simulink library "zero_cross"  (Simulink 6.3)
undefined symbols (not defined in the file): a, b, bits_to_symb_do, DiscIntNeverNeededParam, do_wait, input_stream_sample, j, lookup_do, offset, sfunpsd2
settings Model: Creator=jon  LastModifiedBy=jwallace  ExtModeAutoUpdateStatusClock=off  StrictBusMsg=None

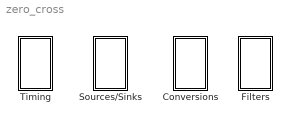
== system zero_cross ==
  Conversions : Subsystem
  Filters : Subsystem
  Sources/Sinks : Subsystem
  "Timing " : Subsystem

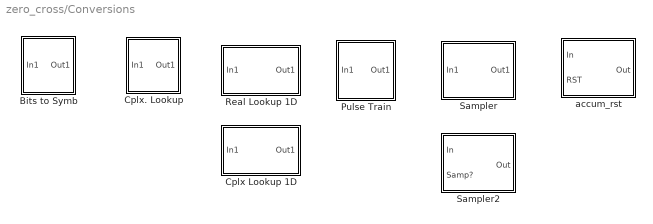
== system zero_cross/Conversions ==
  Bits to Symb : Subsystem
  Cplx Lookup 1D : Subsystem  mask{table=[j -j]}
      mask init:
      | XData = [0:length(table)-1]; YDataRe = real(table); YDataIm = imag(table); XDataEvenlySpacing=1;
  Cplx. Lookup : Subsystem  mask{table=[-1 1]}
      mask help: Does a discrete lookup table.
      mask Help: The table variable has one entry per possible input index.  Note that it is defined to be zero indexed (0 maps to the first table entry, 1 to the second, etc.).
  Pulse Train : Subsystem  mask{period=10}
      mask prompts: period "Period (samples)"
      mask help: Samples the incoming signal and makes a pulse train.
      mask Display: disp(sprintf('T=%d', period));
  Real Lookup 1D : Subsystem  mask{table=[-1 -0.5 0.5 1]}
      mask init:
      | XData = [0:length(table)-1]; YData = table; XDataEvenlySpacing=1;
  Sampler : Subsystem  mask{offset=64, samp_period=10}
      mask prompts: offset "Offset (samples)"; samp_period "Sample Period"
      mask Display: disp(sprintf('del=%d, T=%d', offset, samp_period));
  Sampler2 : Subsystem
  accum_rst : Subsystem

== system zero_cross/Filters ==
  RC FIR Filter : Subsystem  mask{period=10, beta=0.5, root=off, filt_len=128}
      mask prompts: period "Symbol Period"; beta "Roll Off (beta)"; root "Root Filter?"; filt_len "Filter Length (taps)"
      mask init:
      | symb_rate = 1/period; p.fs = symb_rate; p.beta = beta; p.root = root; [h f Ha Hi win] = win_method('rc_filt', p, 1.5*(1+beta)*symb_rate, 1, filt_len, 0); h = h';
      mask Display: plot(f, abs(Ha));
  RECT Filter : Subsystem  AncestorBlock=dsp_blocks/Filters/RC FIR Filter  mask{f0=0.1, f1=0.2, filt_len=64}
      mask prompts: f0 "Low Cutoff (0=LPF)"; f1 "Hi Cutoff"; filt_len "Filter Length (taps)"
      mask init:
      | p.x1 = f0; p.x2 = f0; p.x3 = f1; p.x4 = f1; [h f Ha Hi win] = win_method('pw_lin', p, 0.5, 1, filt_len, 1); h = h';
      mask Display: plot(f, abs(Ha));

== system zero_cross/Sources/Sinks ==
  Averaging Power Spectral Density dB : Subsystem  LoadFcn=sfunpsd2([],[],[],'LoadBlock')  StartFcn=sfunpsd2([],[],[],'Start')  mask(Spectrum Analyzer){npts=128, fftpts=512, HowOften=64, sampleT=1, db_range=20}
      mask prompts: npts "Length of buffer:"; fftpts "Number of points for fft:"; HowOften "Plot after how many points:"; sampleT "Sample time:"; db_range "dB Range:"
      mask help: Spectrum analyzer using graph window.
      mask init:
      | ts=sampleT(1); if length(sampleT) > 1, offset = sampleT(2);, else, offset = 0; end
      settings: CopyFcn=sfunpsd2([],[],[],'CopyBlock')  DeleteFcn=sfunpsd2([],[],[],'DeleteBlock')  NameChangeFcn=sfunpsd2([],[],[],'NameChange')
      mask Help: This block when hooked to the output of a system displays the frequency content of the buffer in the graph window. For more see the M-file sfunpsd.
      mask Display: plot(0,0,100,100,[11,92,92,11,11],[90,90,40,40,90],[82,76,65,57,51,44,35,30,25,20],[65,62,59,63,66,66,67,70,55,50])
  Input Stream : Subsystem  mask{period=10, width=1, fname=data.mat}
      mask prompts: fname "Data Filename"
      mask help: Input Stream: Reads binary data from an input file. Outputs a new value once per period. Width allows you to multiplex output.
      mask init:
      | load(fname); N = floor(length(data)/width); data = reshape(data(1:N*width),width,N);
      mask Help: The function loads the binary data from file fname, which should have a single vector called "data".  The output of the block is updated once every T=width*period.
      mask Display: disp(sprintf('file=%s\nT=%g w=%d', fname, period, width))

== system zero_cross/Timing  ==
  PLL : Subsystem  mask{freq=0.1, freq_out=0.1, phi=0, amp=1, xi=1, K=2, T=200}
      mask prompts: freq "Input Frequency"; freq_out "Output Frequency"; phi "Output Phase"; amp "Output Amplitude"; xi "Damping Factor"; K "Loop Gain"; T "Loop Time Constant (samples)"
      mask help: Implements a phase locked loop (PLL).
      mask init:
      | [a, b, tau1, tau2, Kout] = loop_filter1(T, xi, K);
      mask Display: disp(sprintf('fin=%g fout=%g\nxi=%g Tl=%g\nphi=%g  amp=%g',freq,freq_out,xi,T,phi,amp));
  Real-Time : Subsystem  mask{scale=1}
      mask prompts: scale "Scale Factor"
      mask help: This block slows down a simulation so sample time is some fraction of the real time.
      mask Display: disp('RT');

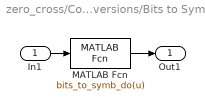
== system zero_cross/Conversions/Bits to Symb ==
  In1 : Inport
  MATLAB Fcn : MATLABFcn  MATLABFcn=bits_to_symb_do(u)  OutputDimensions=1
  Out1 : Outport
  wires:
  MATLAB Fcn/1 -> Out1/1
  In1/1 -> MATLAB Fcn/1

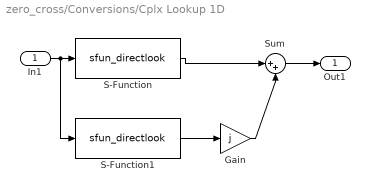
== system zero_cross/Conversions/Cplx Lookup 1D ==
  In1 : Inport
  Gain : Gain  Gain=j  SaturateOnIntegerOverflow=on
  S-Function : S-Function  FunctionName=sfun_directlook  Parameters=XData, YDataRe, XDataEvenlySpacing
  S-Function1 : S-Function  FunctionName=sfun_directlook  Parameters=XData, YDataIm, XDataEvenlySpacing
  Sum : Sum  Inputs=|++  SaturateOnIntegerOverflow=on  InputSameDT=on
  Out1 : Outport
  wires:
  In1/1 -> S-Function1/1, S-Function/1
  S-Function/1 -> Sum/1
  Gain/1 -> Sum/2
  Sum/1 -> Out1/1
  S-Function1/1 -> Gain/1

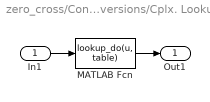
== system zero_cross/Conversions/Cplx. Lookup ==
  In1 : Inport
  MATLAB Fcn : MATLABFcn  MATLABFcn=lookup_do(u, table)  OutputSignalType=complex
  Out1 : Outport
  wires:
  MATLAB Fcn/1 -> Out1/1
  In1/1 -> MATLAB Fcn/1

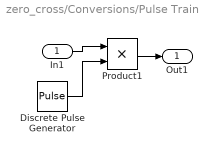
== system zero_cross/Conversions/Pulse Train ==
  In1 : Inport
  Discrete Pulse Generator : DiscretePulseGenerator  Period=period
  Product1 : Product  SaturateOnIntegerOverflow=on  RndMeth=Zero
  Out1 : Outport
  wires:
  Product1/1 -> Out1/1
  In1/1 -> Product1/1
  Discrete Pulse Generator/1 -> Product1/2

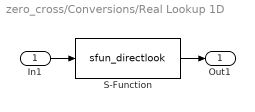
== system zero_cross/Conversions/Real Lookup 1D ==
  In1 : Inport
  S-Function : S-Function  FunctionName=sfun_directlook  Parameters=XData, YData, XDataEvenlySpacing
  Out1 : Outport
  wires:
  S-Function/1 -> Out1/1
  In1/1 -> S-Function/1

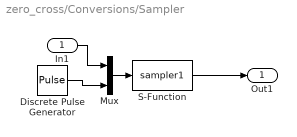
== system zero_cross/Conversions/Sampler ==
  In1 : Inport
  Discrete Pulse Generator : DiscretePulseGenerator  Period=samp_period  PhaseDelay=offset
  Mux : Mux  Inputs=2
  S-Function : S-Function  FunctionName=sampler1
  Out1 : Outport
  wires:
  S-Function/1 -> Out1/1
  Mux/1 -> S-Function/1
  In1/1 -> Mux/1
  Discrete Pulse Generator/1 -> Mux/2

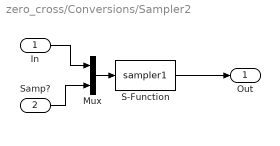
== system zero_cross/Conversions/Sampler2 ==
  In : Inport
  Samp? : Inport  Port=2
  Mux : Mux  Inputs=2
  S-Function : S-Function  FunctionName=sampler1
  Out : Outport
  wires:
  Samp?/1 -> Mux/2
  In/1 -> Mux/1
  Mux/1 -> S-Function/1
  S-Function/1 -> Out/1

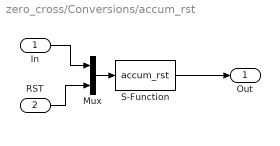
== system zero_cross/Conversions/accum_rst ==
  In : Inport
  RST : Inport  Port=2
  Mux : Mux  Inputs=2
  S-Function : S-Function  FunctionName=accum_rst
  Out : Outport
  wires:
  S-Function/1 -> Out/1
  Mux/1 -> S-Function/1
  In/1 -> Mux/1
  RST/1 -> Mux/2

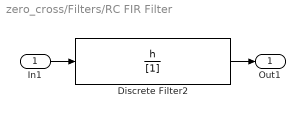
== system zero_cross/Filters/RC FIR Filter ==
  In1 : Inport
  Discrete Filter2 : DiscreteFilter  Numerator=h  Denominator=[1]
  Out1 : Outport
  wires:
  Discrete Filter2/1 -> Out1/1
  In1/1 -> Discrete Filter2/1

== system zero_cross/Filters/RECT Filter ==
  In1 : Inport
  Discrete Filter2 : DiscreteFilter  Numerator=h  Denominator=[1]
  Out1 : Outport
  wires:
  In1/1 -> Discrete Filter2/1
  Discrete Filter2/1 -> Out1/1

== system zero_cross/Sources/Sinks/Averaging Power Spectral Density dB ==
  input signal : Inport
  sfunpsd2 : S-Function  LoadFcn=sfunpsd2([],[],[],'LoadBlock')  StartFcn=sfunpsd2([],[],[],'Start')  FunctionName=sfunpsd2  Parameters=fftpts,npts,HowOften,offset,ts,1,db_range
      settings: CopyFcn=sfunpsd2([],[],[],'CopyBlock')  DeleteFcn=sfunpsd2([],[],[],'DeleteBlock')  NameChangeFcn=sfunpsd2([],[],[],'NameChange')
  wires:
  input signal/1 -> sfunpsd2/1

== system zero_cross/Sources/Sinks/Input Stream ==
  Clock : Clock
  MATLAB Fcn : MATLABFcn  MATLABFcn=input_stream_sample(u, data, period, width)  OutputDimensions=width  Output1D=off
  Out1 : Outport
  wires:
  MATLAB Fcn/1 -> Out1/1
  Clock/1 -> MATLAB Fcn/1

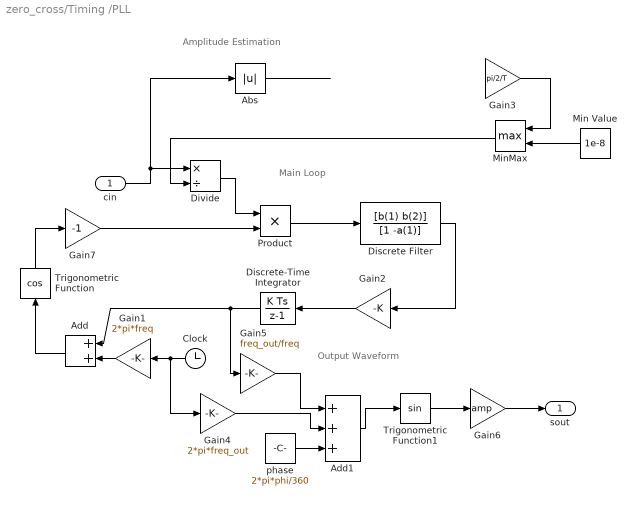
== system zero_cross/Timing /PLL ==
  note: Output Waveform
  note: Main Loop
  note: Amplitude Estimation
  cin : Inport
  Abs : Abs
  Add : Sum  Orientation=left  OutScaling=2^-10
  Add1 : Sum  Inputs=+++  OutScaling=2^-10
  Clock : Clock
  Discrete Filter : DiscreteFilter  Numerator=[b(1) b(2)]  Denominator=[1 -a(1)]
  Discrete-Time Integrator : DiscreteIntegrator  Orientation=left  gainval=1  ICPrevOutput=DiscIntNeverNeededParam  ICPrevScaledInput=DiscIntNeverNeededParam
  Divide : Product  Inputs=*/  OutScaling=2^-10
  Gain1 : Gain  Orientation=left  Gain=2*pi*freq
  Gain2 : Gain  Orientation=left  Gain=-K
  Gain3 : Gain  Gain=pi/2/T
  Gain4 : Gain  Gain=2*pi*freq_out
  Gain5 : Gain  Gain=freq_out/freq
  Gain6 : Gain  Gain=amp
  Gain7 : Gain  Gain=-1
  Min Value : Constant  Orientation=left  Value=1e-8
  MinMax : MinMax  Orientation=left  Function=max  Inputs=2
  Product : Product  RndMeth=Zero
  Trigonometric Function : Trigonometry  Orientation=up  Operator=cos
  Trigonometric Function1 : Trigonometry
  phase : Constant  Value=2*pi*phi/360
  sout : Outport
  wires:
  Trigonometric Function1/1 -> Gain6/1
  Add1/1 -> Trigonometric Function1/1
  Gain5/1 -> Add1/1
  Gain4/1 -> Add1/2
  Min Value/1 -> MinMax/2
  MinMax/1 -> Divide/2
  Gain3/1 -> MinMax/1
  Divide/1 -> Product/1
  cin/1 -> Divide/1, Abs/1
  ? -> Gain3/1
  Abs/1 -> ?
  Discrete Filter/1 -> Gain2/1
  Gain2/1 -> Discrete-Time Integrator/1
  Trigonometric Function/1 -> Gain7/1
  Add/1 -> Trigonometric Function/1
  Discrete-Time Integrator/1 -> Gain5/1, Add/1
  Gain1/1 -> Add/2
  Clock/1 -> Gain4/1, Gain1/1
  Product/1 -> Discrete Filter/1
  Gain6/1 -> sout/1
  Gain7/1 -> Product/2
  phase/1 -> Add1/3

== system zero_cross/Timing /Real-Time ==
  Clock : Clock
  MATLAB Fcn : MATLABFcn  Description=do_wait  MATLABFcn=do_wait(u, scale)  OutputDimensions=0
  wires:
  Clock/1 -> MATLAB Fcn/1
